simulink model "dac_point_generator"  (R2021a)
settings: Solver=VariableStepAuto  StartTime=0.0  StopTime=10.0  RelTol=1e-3
libraries: dspxfrm3 x1
settings Model: Creator=Ayush  LastModifiedBy=Sankalp

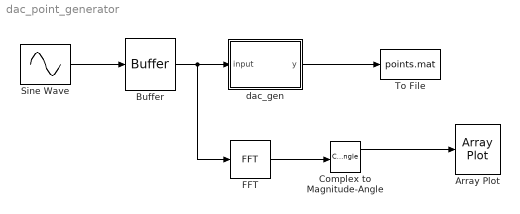
== system dac_point_generator ==
  Array Plot : ArrayPlot  WindowPosition=[-1106.000000,306.000000,800.000000,500.000000,]  YLimits=[-47.401148229206456,426.6236230872108]  DefaultConfigurationName=dsp.scopes.ArrayPlotBlockSpecification
  Buffer : Buffer  N=10000  OutputFrames=off
  Complex to Magnitude-Angle : ComplexToMagnitudeAngle
  FFT : dspxfrm3/FFT  FFTImplementation=Auto  CompMethod=Table lookup  TableOpt=NEW  TableOptActive=Speed  BitRevOrder=off  Normalize=off  InheritFFTLength=on  FFTLength=64  WrapInput=on  roundingMode=Floor  overflowMode=off  firstCoeffDataTypeStr=Inherit: Same word length as input  firstCoeffLastDataTypeStr=Inherit: Same word length as input  outputMin=[]  outputMax=[]
  Sine Wave : Sin  Frequency=6308.3180412  SampleTime=0.0001
  To File : ToFile  Filename=points.mat  SaveFormat=Timeseries
  dac_gen : MATLAB Function  TreatAsAtomicUnit=on
  wires:
  Sine Wave/1 -> Buffer/1
  Buffer/1 -> FFT/1, dac_gen/1(input)
  dac_gen/1(y) -> To File/1
  FFT/1 -> Complex to Magnitude-Angle/1
  Complex to Magnitude-Angle/1 -> Array Plot/1

== matlab function dac_point_generator/dac_gen ==
  data: input input; y output
function y = fcn(input)
    input = input';
    points_btw_two_samples = 10;
    total_point = length(input)*points_btw_two_samples;
    dac_arr = zeros(1, total_point);
    dac_arr_index = 1;

    for i = 1:length(input)-1
        dac_arr(dac_arr_index) = input(i);
        dac_arr_index = dac_arr_index + 1;
        for j = 1:(points_btw_two_samples-1)
            slope = (input(i+1) - input(i));
            dac_arr(dac_arr_index) = input(i) + (slope/(points_btw_two_samples-j));
            dac_arr_index = dac_arr_index + 1;
        end
    end

%     fileID = fopen('sine_dac_points_gen.txt','w');
%     fprintf(fileID,'%f\n',dac_arr);
%     fclose(fileID);

y = dac_arr;
